simulink model "IQ_demod"  (R2025b)
settings: Solver=VariableStepAuto  StartTime=0.0  StopTime=10.0  RelTol=1e-3
libraries: simrfV2elements x4, simrfV2sources1 x2, simrfV2util1 x1
settings Model: Creator=isaacahn  LastModifiedBy=isaacahn

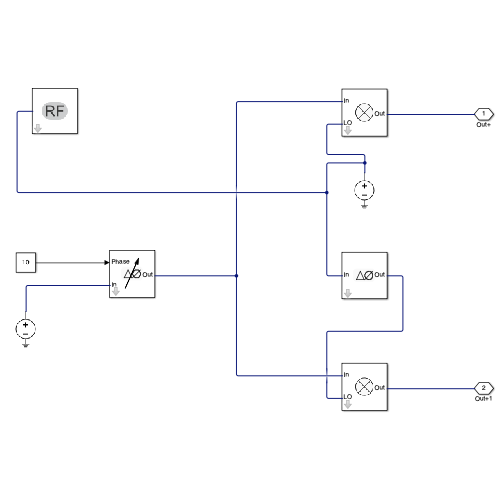
[thumbnail: Simulink's stored preview of the top-level diagram]
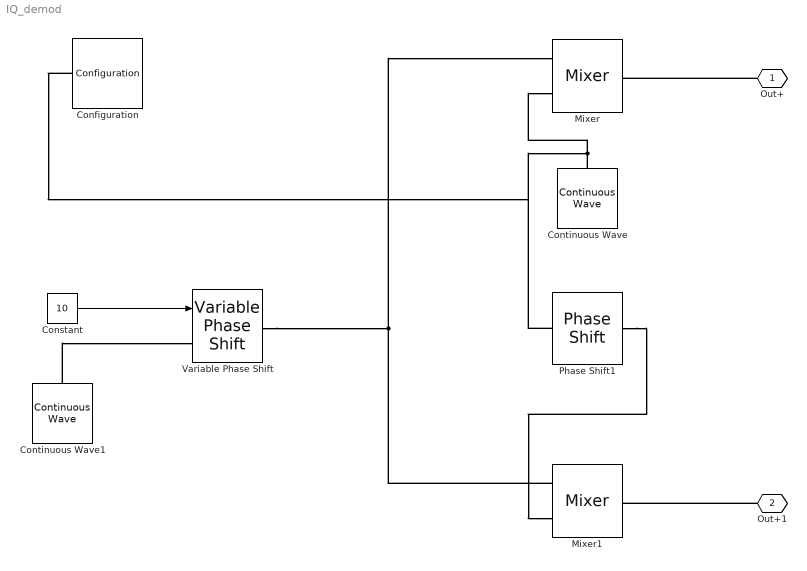
== system IQ_demod ==
  Configuration : simrfV2util1/Configuration  AutoFreq=on  Tones=[] Hz  Harmonics=[]  NormalizeCarrierPower=on  SolverType=Auto  UseCCode=on  StepSize=1e-6 s  AddNoise=on  defaultRNG=on  Seed=0  Temperature=25 C  SolverDelFlag=0  AbsTol=1e-6  RelTol=1e-3  MaxIter=10  ErrorEstimationType=2-norm over all variables  EnableInterpFilter=on  HiddenFIRfilterControllerParam=off  SmallSignalApprox=off  AllSimFreqs=on  SimFreqs=[] Hz  SimFreqsInternal=[]  SamplesPerFrame=1
  Constant : Constant  Value=10
  Continuous Wave : simrfV2sources1/Continuous Wave  CWSourceType=Ideal voltage  Z0=0  IVoltage=0 V  ICurrent=0 A  MagPower=0 W  QVoltage=0 V  QCurrent=0 A  AnglePower=0  CarrierFreq=2.4 GHz  AddPhaseNoise=off  PhaseNoiseOffset=1  PhaseNoiseLevel=-Inf  AutoImpulseLength=on  ImpulseLength=1e-10 s  InternalGrounding=on
  Continuous Wave1 : simrfV2sources1/Continuous Wave  CWSourceType=Ideal voltage  Z0=0  IVoltage=0 V  ICurrent=0 A  MagPower=0 W  QVoltage=0 V  QCurrent=0 A  AnglePower=0  CarrierFreq=2.4 GHz  AddPhaseNoise=off  PhaseNoiseOffset=1  PhaseNoiseLevel=-Inf  AutoImpulseLength=on  ImpulseLength=1e-10 s  InternalGrounding=on
  Mixer : simrfV2elements/Mixer  classname=mixer  Source_linear_gain=Available power gain  linear_gain=0 dB  Zin=50  Zout=50  ZLO=inf  Source_Poly=Even and odd order  Poly_Coeffs=[0 1]  IPType=Output  IP2=Inf dBm  IP3=Inf dBm  P1dB=Inf dBm  Psat=Inf dBm  Gcomp=Inf dBm  NF=0  InternalGrounding=on
  Mixer1 : simrfV2elements/Mixer  classname=mixer  Source_linear_gain=Available power gain  linear_gain=0 dB  Zin=50  Zout=50  ZLO=inf  Source_Poly=Even and odd order  Poly_Coeffs=[0 1]  IPType=Output  IP2=Inf dBm  IP3=Inf dBm  P1dB=Inf dBm  Psat=Inf dBm  Gcomp=Inf dBm  NF=0  InternalGrounding=on
  Phase Shift1 : simrfV2elements/Phase Shift  PhaseShift=90 deg  InternalGrounding=on  PCBConvertable=on  PCBObjDesign={'design(phaseShifter,<DesignFreq>,''PhaseShift'',convert2Deg(<PhaseShift>,<PhaseShift_unit>))'}  PCBObjAllowed={{'phaseShifter'}}  PCBObjReroute={cell(1,0)}
  Variable Phase Shift : simrfV2elements/Variable Phase Shift  classname=varphase  PhaseShift_unit=deg  SparamZ0=50  InternalGrounding=on
  Out+ : PMIOPort  Tag=PMCPort  Side=Right
  Out+1 : PMIOPort  Tag=PMCPort  Port=2  Side=Right
  wires:
  Constant/1 -> Variable Phase Shift/1
  connections:
  Continuous Wave/LConn1 -- Phase Shift1/LConn1 -- Configuration/LConn1 -- Mixer/LConn2
  Phase Shift1/RConn1 -- Mixer1/LConn2
  Variable Phase Shift/RConn1 -- Mixer/LConn1 -- Mixer1/LConn1
  Continuous Wave1/LConn1 -- Variable Phase Shift/LConn1
  Out+/RConn1 -- Mixer/RConn1
  Out+1/RConn1 -- Mixer1/RConn1
